simulink subsystem "drone_navigation"  (R2023a)
settings: Solver=VariableStepAuto  StartTime=0.0  StopTime=10.0  RelTol=1e-3
undefined symbols (not defined in the file or in its folder): Discrete, param, Time
libraries: dspfdesign x20, sharedTrackingLibrary x1, ctrlSharedLib x1, dspmtrx3 x1, simulink_extras x1
settings Model: Creator=timme  LastModifiedBy=timme

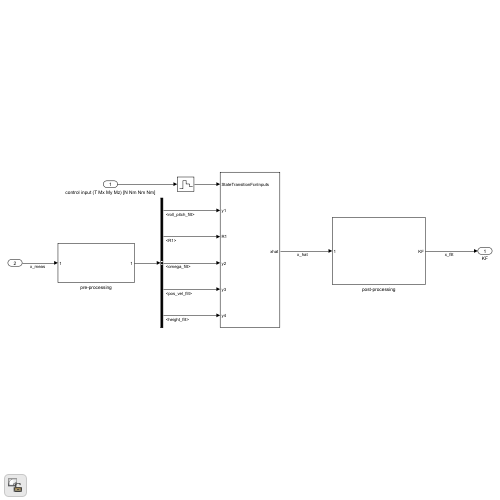
[thumbnail: Simulink's stored preview of the top-level diagram]
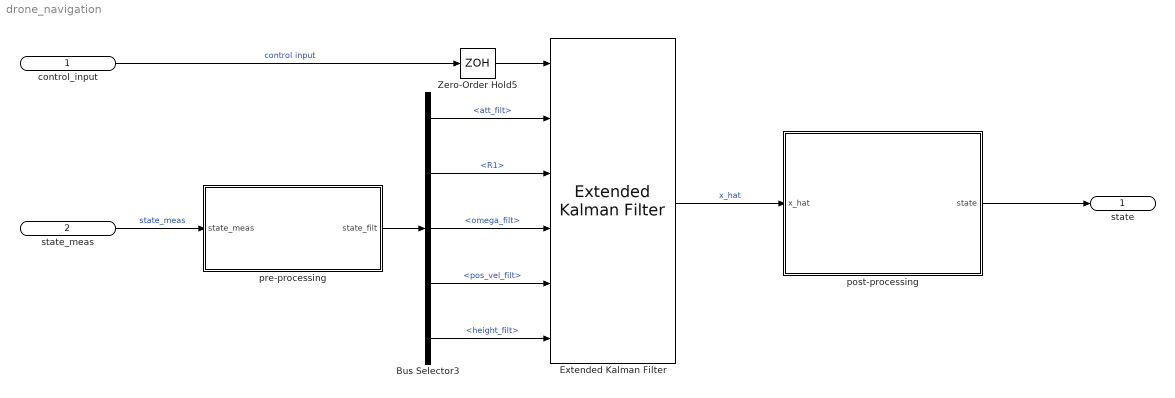
== system drone_navigation ==
  control_input : Inport  PortDimensions=4
  state_meas : Inport  Port=2  PortDimensions=14
  Bus Selector3 : BusSelector  OutputSignals=att_filt,R1,omega_filt,pos_vel_filt,height_filt
  Extended Kalman Filter : sharedTrackingLibrary/Extended Kalman Filter  StateTransitionFcn=stateTransition  HasStateTransitionJacobianFcn=off  HasAdditiveProcessNoise=Additive  ProcessNoise=diag([1*ones(1,6) [1 1 0.01] [0.1 0.1 0.1]])  HasTimeVaryingProcessNoise=off  HasStateTransitionFcnExtraArgument=1  InitialState=zeros(12,1)  InitialStateCovariance=zeros(12)  MeasurementFcn1=accelerometer_model  HasMeasurementJacobianFcn1=off  HasMeasurementEnablePort1=off  HasAdditiveMeasurementNoise1=Additive  MeasurementNoise1=diag([1 1])  HasTimeVaryingMeasurementNoise1=on  HasMeasurementFcnExtraArgument1=0  HasMeasurementWrapping1=off  MeasurementFcn2=gyrometer_model  HasMeasurementJacobianFcn2=off  HasMeasurementEnablePort2=off  HasAdditiveMeasurementNoise2=Additive  MeasurementNoise2=diag([1 1 1])  HasTimeVaryingMeasurementNoise2=off  HasMeasurementFcnExtraArgument2=0  HasMeasurementWrapping2=off  MeasurementFcn3=GPS_model  HasMeasurementJacobianFcn3=off  HasMeasurementEnablePort3=off  HasAdditiveMeasurementNoise3=Additive  MeasurementNoise3=diag([0.001 0.001 0.001 0.001 0.001 0.001])  HasTimeVaryingMeasurementNoise3=off  HasMeasurementFcnExtraArgument3=0  HasMeasurementWrapping3=off  MeasurementFcn4=Barometer_model  HasMeasurementJacobianFcn4=off  HasMeasurementEnablePort4=off  HasAdditiveMeasurementNoise4=Additive  MeasurementNoise4=0.001  HasTimeVaryingMeasurementNoise4=off  HasMeasurementFcnExtraArgument4=0  HasMeasurementWrapping4=off  MeasurementFcn5=myMeasurementFcn  HasMeasurementJacobianFcn5=off  HasMeasurementEnablePort5=off  HasAdditiveMeasurementNoise5=Additive  MeasurementNoise5=1  HasTimeVaryingMeasurementNoise5=off  HasMeasurementFcnExtraArgument5=0  HasMeasurementWrapping5=off  EnableMultirate=off  StateTransitionFcnSampleTime=0.001  MeasurementFcn1SampleTime=0.001  MeasurementFcn2SampleTime=0.001  MeasurementFcn3SampleTime=0.1  MeasurementFcn4SampleTime=0.01  MeasurementFcn5SampleTime=1  UseCurrentEstimator=on  OutputStateCovariance=off  DataType=double  SampleTime=0.001  NumberOfMeasurements=4
  Zero-Order Hold5 : ZeroOrderHold  SampleTime=0.001
  post-processing : Subsystem  Description=Post-processing is performed on the estimated state through a low pass filter to further smoothen the signals
  pre-processing : Subsystem  Description=|
      | Pre-processing of the measured variables through filtering the high-frequency noise from the signals.
      | A Kalman filter is used to estimate the pitch and roll angles from the IMU measurements
  state : Outport  PortDimensions=12
  wires:
  Zero-Order Hold5/1 -> Extended Kalman Filter/1
  state_meas/1 -> pre-processing/1(state_meas)  "state_meas"
  control_input/1 -> Zero-Order Hold5/1  "control input"
  pre-processing/1(state_filt) -> Bus Selector3/1
  Bus Selector3/1 -> Extended Kalman Filter/2  "<att_filt>"
  Bus Selector3/3 -> Extended Kalman Filter/4  "<omega_filt>"
  Bus Selector3/4 -> Extended Kalman Filter/5  "<pos_vel_filt>"
  Bus Selector3/5 -> Extended Kalman Filter/6  "<height_filt>"
  Bus Selector3/2 -> Extended Kalman Filter/3  "<R1>"
  Extended Kalman Filter/1 -> post-processing/1(x_hat)  "x_hat"
  post-processing/1(state) -> state/1

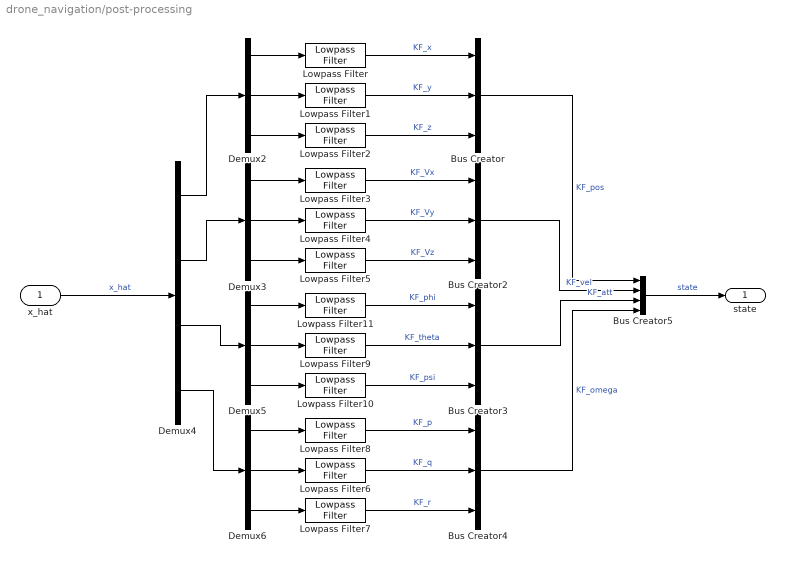
== system drone_navigation/post-processing ==
  x_hat : Inport  PortDimensions=12
  Bus Creator{,2..4} (4 alike) : BusCreator  Inputs=3
  Bus Creator5 : BusCreator  Inputs=4
  Demux{2..3,5..6} (4 alike) : Demux  Outputs=3
  Demux4 : Demux
  Lowpass Filter{,1..5,9..11} (9 alike) : dspfdesign/Lowpass Filter  FilterType=IIR  DesignForMinimumOrder=on  FilterOrder=50  PassbandFrequency=1  StopbandFrequency=499  PassbandRipple=0.1  StopbandAttenuation=50  SampleRateMode=Specify on dialog  SampleRate=1000  SimulateUsing=Interpreted execution  roundingMode=Floor  coeffsDataTypeStr=fixdt(1,16)
  Lowpass Filter6 : dspfdesign/Lowpass Filter  FilterType=IIR  DesignForMinimumOrder=on  FilterOrder=50  PassbandFrequency=1  StopbandFrequency=100  PassbandRipple=0.1  StopbandAttenuation=45  SampleRateMode=Specify on dialog  SampleRate=1000  SimulateUsing=Interpreted execution  roundingMode=Floor  coeffsDataTypeStr=fixdt(1,16)
  Lowpass Filter7 : dspfdesign/Lowpass Filter  FilterType=IIR  DesignForMinimumOrder=on  FilterOrder=50  PassbandFrequency=1  StopbandFrequency=100  PassbandRipple=0.1  StopbandAttenuation=45  SampleRateMode=Specify on dialog  SampleRate=1000  SimulateUsing=Interpreted execution  roundingMode=Floor  coeffsDataTypeStr=fixdt(1,16)
  Lowpass Filter8 : dspfdesign/Lowpass Filter  FilterType=IIR  DesignForMinimumOrder=on  FilterOrder=50  PassbandFrequency=1  StopbandFrequency=100  PassbandRipple=0.1  StopbandAttenuation=45  SampleRateMode=Specify on dialog  SampleRate=1000  SimulateUsing=Interpreted execution  roundingMode=Floor  coeffsDataTypeStr=fixdt(1,16)
  state : Outport  PortDimensions=12
  wires:
  x_hat/1 -> Demux4/1  "x_hat"
  Lowpass Filter10/1 -> Bus Creator3/3  "KF_psi"
  Demux5/3 -> Lowpass Filter10/1
  Bus Creator5/1 -> state/1  "state"
  Lowpass Filter4/1 -> Bus Creator2/2  "KF_Vy"
  Demux6/3 -> Lowpass Filter7/1
  Lowpass Filter8/1 -> Bus Creator4/1  "KF_p"
  Demux6/1 -> Lowpass Filter8/1
  Demux5/2 -> Lowpass Filter9/1
  Bus Creator2/1 -> Bus Creator5/2  "KF_vel"
  Demux5/1 -> Lowpass Filter11/1
  Lowpass Filter7/1 -> Bus Creator4/3  "KF_r"
  Demux6/2 -> Lowpass Filter6/1
  Lowpass Filter11/1 -> Bus Creator3/1  "KF_phi"
  Bus Creator4/1 -> Bus Creator5/4  "KF_omega"
  Lowpass Filter2/1 -> Bus Creator/3  "KF_z"
  Demux4/1 -> Demux2/1
  Demux4/3 -> Demux5/1
  Demux3/2 -> Lowpass Filter4/1
  Lowpass Filter6/1 -> Bus Creator4/2  "KF_q"
  Demux4/2 -> Demux3/1
  Demux3/3 -> Lowpass Filter5/1
  Lowpass Filter9/1 -> Bus Creator3/2  "KF_theta"
  Bus Creator3/1 -> Bus Creator5/3  "KF_att"
  Lowpass Filter5/1 -> Bus Creator2/3  "KF_Vz"
  Bus Creator/1 -> Bus Creator5/1  "KF_pos"
  Lowpass Filter3/1 -> Bus Creator2/1  "KF_Vx"
  Demux2/3 -> Lowpass Filter2/1
  Demux4/4 -> Demux6/1
  Demux2/1 -> Lowpass Filter/1
  Demux2/2 -> Lowpass Filter1/1
  Lowpass Filter1/1 -> Bus Creator/2  "KF_y"
  Lowpass Filter/1 -> Bus Creator/1  "KF_x"
  Demux3/1 -> Lowpass Filter3/1

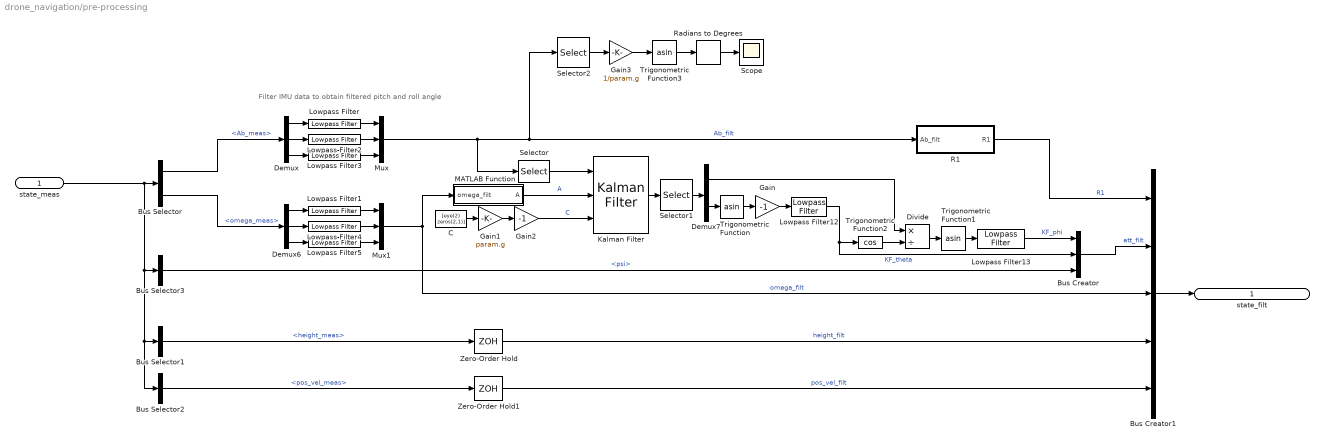
== system drone_navigation/pre-processing ==
  note: Filter IMU data to obtain filtered pitch and roll angle
  state_meas : Inport  PortDimensions=14
  Bus Creator : BusCreator  Inputs=3
  Bus Creator1 : BusCreator  Inputs=5
  Bus Selector : BusSelector  OutputSignals=Ab_meas,omega_meas
  Bus Selector1 : BusSelector  OutputSignals=height_meas
  Bus Selector2 : BusSelector  OutputSignals=pos_vel_meas
  Bus Selector3 : BusSelector  OutputSignals=psi
  C : Constant  Value=[eye(2) zeros(2,1)]
  Demux : Demux  Outputs=3
  Demux6 : Demux  Outputs=3
  Demux7 : Demux  Outputs=2
  Divide : Product  Inputs=*/
  Gain : Gain  Gain=-1
  Gain1 : Gain  Gain=param.g
  Gain2 : Gain  Gain=-1
  Gain3 : Gain  Gain=1/param.g
  Kalman Filter : ctrlSharedLib/Kalman Filter  TimeDomain=Discrete-Time  UseCurrentEstimator=on  ModelSource=Input port  ModelSourceVariable=ss(0.95,1,1,0,1)  A=0.95  B=1  C=1  D=0  NumberOfStates=3  NumberOfInputs=1  NumberOfOutputs=2  InitialEstimateSource=Dialog  X0=0  P0=1  UseK=off  UseGH=off  NumberOfProcessNoiseInputs=1  G=eye(3)  TimeInvariantG=on  H=ones(2,1)  TimeInvariantH=on  Q=100  TimeInvariantQ=on  R=0.0001  TimeInvariantR=on  N=0  TimeInvariantN=on  AddInputPort=off  AddEnablePort=off  OutputEstimatedY=off  OutputP=off  Ts=0.001
  Lowpass Filter : dspfdesign/Lowpass Filter  FilterType=IIR  DesignForMinimumOrder=on  FilterOrder=50  PassbandFrequency=1  StopbandFrequency=499  PassbandRipple=0.1  StopbandAttenuation=80  SampleRateMode=Specify on dialog  SampleRate=1000  SimulateUsing=Interpreted execution  roundingMode=Floor  coeffsDataTypeStr=fixdt(1,16)
  Lowpass Filter1 : dspfdesign/Lowpass Filter  FilterType=IIR  DesignForMinimumOrder=on  FilterOrder=50  PassbandFrequency=25  StopbandFrequency=499  PassbandRipple=0.1  StopbandAttenuation=80  SampleRateMode=Specify on dialog  SampleRate=1000  SimulateUsing=Interpreted execution  roundingMode=Floor  coeffsDataTypeStr=fixdt(1,16)
  Lowpass Filter12 : dspfdesign/Lowpass Filter  FilterType=IIR  DesignForMinimumOrder=on  FilterOrder=50  PassbandFrequency=5  StopbandFrequency=60  PassbandRipple=0.1  StopbandAttenuation=45  SampleRateMode=Specify on dialog  SampleRate=1000  SimulateUsing=Interpreted execution  roundingMode=Floor  coeffsDataTypeStr=fixdt(1,16)
  Lowpass Filter13 : dspfdesign/Lowpass Filter  FilterType=IIR  DesignForMinimumOrder=on  FilterOrder=50  PassbandFrequency=5  StopbandFrequency=60  PassbandRipple=0.1  StopbandAttenuation=45  SampleRateMode=Specify on dialog  SampleRate=1000  SimulateUsing=Interpreted execution  roundingMode=Floor  coeffsDataTypeStr=fixdt(1,16)
  Lowpass Filter2 : dspfdesign/Lowpass Filter  FilterType=IIR  DesignForMinimumOrder=on  FilterOrder=50  PassbandFrequency=1  StopbandFrequency=499  PassbandRipple=0.1  StopbandAttenuation=80  SampleRateMode=Specify on dialog  SampleRate=1000  SimulateUsing=Interpreted execution  roundingMode=Floor  coeffsDataTypeStr=fixdt(1,16)
  Lowpass Filter3 : dspfdesign/Lowpass Filter  FilterType=IIR  DesignForMinimumOrder=on  FilterOrder=50  PassbandFrequency=1  StopbandFrequency=499  PassbandRipple=0.1  StopbandAttenuation=80  SampleRateMode=Specify on dialog  SampleRate=1000  SimulateUsing=Interpreted execution  roundingMode=Floor  coeffsDataTypeStr=fixdt(1,16)
  Lowpass Filter4 : dspfdesign/Lowpass Filter  FilterType=IIR  DesignForMinimumOrder=on  FilterOrder=50  PassbandFrequency=25  StopbandFrequency=499  PassbandRipple=0.1  StopbandAttenuation=80  SampleRateMode=Specify on dialog  SampleRate=1000  SimulateUsing=Interpreted execution  roundingMode=Floor  coeffsDataTypeStr=fixdt(1,16)
  Lowpass Filter5 : dspfdesign/Lowpass Filter  FilterType=IIR  DesignForMinimumOrder=on  FilterOrder=50  PassbandFrequency=25  StopbandFrequency=499  PassbandRipple=0.1  StopbandAttenuation=80  SampleRateMode=Specify on dialog  SampleRate=1000  SimulateUsing=Interpreted execution  roundingMode=Floor  coeffsDataTypeStr=fixdt(1,16)
  MATLAB Function : MATLAB Function  TreatAsAtomicUnit=on
  Mux : Mux  Inputs=3
  Mux1 : Mux  Inputs=3
  R1 : Subsystem
  Radians to Degrees : simulink_extras/Transformations/Radians to Degrees
  Scope : Scope
  Selector : Selector  InputPortWidth=3  IndexOptions=Index vector (dialog)  Indices=[1 2]  OutputSizes=1
  Selector1 : Selector  InputPortWidth=3  IndexOptions=Index vector (dialog)  Indices=[2 1]  OutputSizes=1
  Selector2 : Selector  InputPortWidth=3  IndexOptions=Index vector (dialog)  Indices=[1]  OutputSizes=1
  Trigonometric Function : Trigonometry  Operator=asin
  Trigonometric Function1 : Trigonometry  Operator=asin  OutputSignalType=real
  Trigonometric Function2 : Trigonometry  Operator=cos
  Trigonometric Function3 : Trigonometry  Operator=asin
  Zero-Order Hold : ZeroOrderHold  SampleTime=0.001
  Zero-Order Hold1 : ZeroOrderHold  SampleTime=0.001
  state_filt : Outport
  wires:
  Radians to Degrees/1 -> Scope/1
  Trigonometric Function3/1 -> Radians to Degrees/1
  Selector2/1 -> Gain3/1
  Gain3/1 -> Trigonometric Function3/1
  Bus Selector3/1 -> Bus Creator/3  "<psi>"
  Gain2/1 -> Kalman Filter/3  "C"
  Gain1/1 -> Gain2/1
  Demux/2 -> Lowpass Filter2/1
  R1/1(R1) -> Bus Creator1/1  "R1"
  Mux/1 -> Selector/1, Selector2/1, R1/1(Ab_filt)  "Ab_filt"
  Zero-Order Hold/1 -> Bus Creator1/4  "height_filt"
  Zero-Order Hold1/1 -> Bus Creator1/5  "pos_vel_filt"
  Bus Selector2/1 -> Zero-Order Hold1/1  "<pos_vel_meas>"
  Bus Creator/1 -> Bus Creator1/2  "att_filt"
  Bus Selector1/1 -> Zero-Order Hold/1  "<height_meas>"
  Bus Creator1/1 -> state_filt/1
  Mux1/1 -> Bus Creator1/3, MATLAB Function/1(omega_filt)  "omega_filt"
  Demux/1 -> Lowpass Filter/1
  Demux6/2 -> Lowpass Filter4/1
  Lowpass Filter/1 -> Mux/1
  Lowpass Filter5/1 -> Mux1/3
  Demux6/3 -> Lowpass Filter5/1
  Lowpass Filter2/1 -> Mux/2
  Demux/3 -> Lowpass Filter3/1
  Lowpass Filter1/1 -> Mux1/1
  Lowpass Filter4/1 -> Mux1/2
  Lowpass Filter3/1 -> Mux/3
  Demux6/1 -> Lowpass Filter1/1
  state_meas/1 -> Bus Selector1/1, Bus Selector2/1, Bus Selector3/1, Bus Selector/1
  Lowpass Filter13/1 -> Bus Creator/1  "KF_phi"
  Demux7/1 -> Divide/1
  Selector1/1 -> Demux7/1
  Kalman Filter/1 -> Selector1/1
  Trigonometric Function/1 -> Gain/1
  C/1 -> Gain1/1
  Gain/1 -> Lowpass Filter12/1
  Demux7/2 -> Trigonometric Function/1
  Selector/1 -> Kalman Filter/1
  Lowpass Filter12/1 -> Bus Creator/2, Trigonometric Function2/1  "KF_theta"
  Bus Selector/1 -> Demux/1  "<Ab_meas>"
  Bus Selector/2 -> Demux6/1  "<omega_meas>"
  Trigonometric Function2/1 -> Divide/2
  Trigonometric Function1/1 -> Lowpass Filter13/1
  Divide/1 -> Trigonometric Function1/1
  MATLAB Function/1(A) -> Kalman Filter/2  "A"

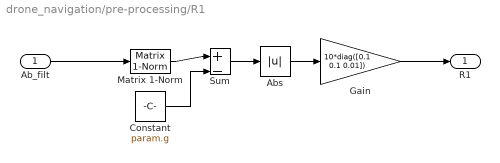
== system drone_navigation/pre-processing/R1 ==
  Ab_filt : Inport
  Abs : Abs  SaturateOnIntegerOverflow=off
  Constant : Constant  Value=param.g
  Gain : Gain  Gain=10*diag([0.1 0.1 0.01])
  Matrix 1-Norm : dspmtrx3/Matrix  1-Norm  roundingMode=Floor  overflowMode=off  outputDataTypeStr=Inherit: Same as accumulator  outputMin=[]  outputMax=[]  outputLastDataTypeStr=Inherit: Same as accumulator
  Sum : Sum  Inputs=|+-
  R1 : Outport
  wires:
  Abs/1 -> Gain/1
  Gain/1 -> R1/1
  Sum/1 -> Abs/1
  Constant/1 -> Sum/2
  Ab_filt/1 -> Matrix 1-Norm/1
  Matrix 1-Norm/1 -> Sum/1

== matlab function drone_navigation/pre-processing/MATLAB Function ==
  data: omega_filt input; A output
function A = fcn(omega_filt)

A = -[0 -omega_filt(int8(3)) omega_filt(int8(2));
    omega_filt(int8(3)) 0 -omega_filt(int8(1));
    -omega_filt(int8(2)) omega_filt(int8(1)) 0 ];
